simulink model "sysob_simulink"  (R2018b)
settings: Solver=VariableStepAuto  StartTime=0.0  StopTime=10.0  RelTol=1e-3
model workspace: external: MAT-File M:\ParaPower\ARL_ParaPower\Validation\MItest.mat (data not in the file)
values from neighbouring files (symbols this model uses):
  htcs = [1500 1500 500 500 500 500 500 500 500 500]    [MItest.mat]
  Ta_vec = [50 50 50 50 50 50 50 50 50 50]    [MItest.mat]
settings Model: Creator=michael.c.fish  LastModifiedBy=michael.c.fish

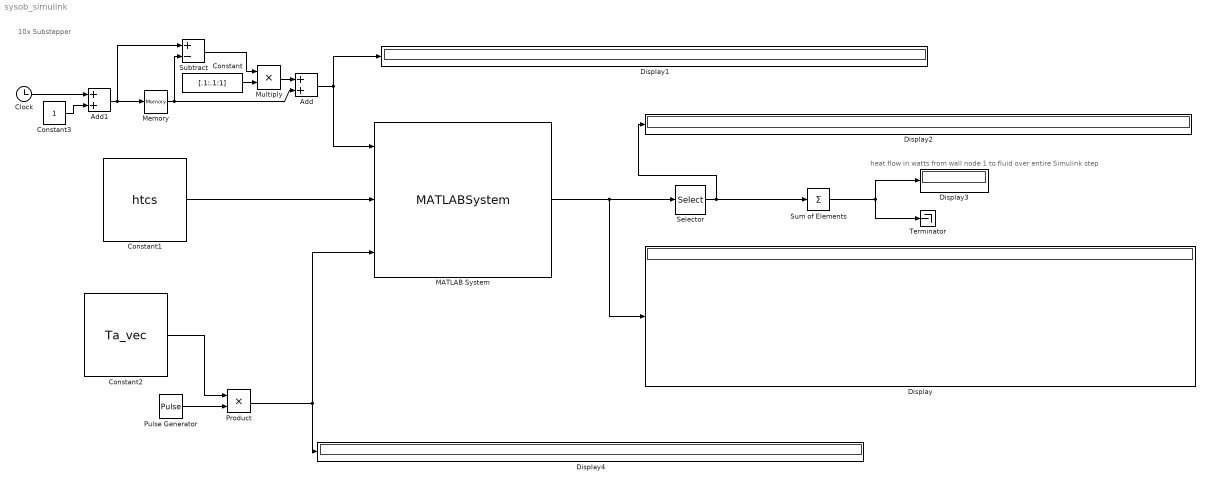
== system sysob_simulink ==
  note: heat flow in watts from wall node 1 to fluid over entire Simulink step
  note: 10x Substepper
  Add : Sum
  Add1 : Sum
  Clock : Clock
  Constant : Constant  Value=[.1:.1:1]  VectorParams1D=off
  Constant1 : Constant  Value=htcs  VectorParams1D=off
  Constant2 : Constant  Value=Ta_vec  VectorParams1D=off
  Constant3 : Constant
  Display{,1..4} (5 alike) : Display
  MATLAB System : MATLABSystem  System=hookPPT  MI=MI  SimulateUsing=Interpreted execution
      mask Type: hookPPT
      mask Display:
      | disp('hookPPT');
      | port_label('input',1,'GlobalTime');
      | port_label('input',2,'htcs');
      | port_label('input',3,'Ta_vec');
      | port_label('output',1,'bdry_watts');
  Memory : Memory
  Multiply : Product
  Product : Product
  Pulse Generator : DiscretePulseGenerator  PulseType=Time based  Period=10  PulseWidth=50
  Selector : Selector  NumberOfDimensions=2  InputPortWidth=3  IndexOptions=Index vector (dialog),Select all  Indices=1,1  OutputSizes=1,1
  Subtract : Sum  Inputs=+-
  Sum of Elements : Sum  Inputs=+
  Terminator : Terminator
  wires:
  Constant1/1 -> MATLAB System/2
  MATLAB System/1 -> Display/1, Selector/1
  Selector/1 -> Sum of Elements/1, Display2/1
  Pulse Generator/1 -> Product/2
  Constant2/1 -> Product/1
  Product/1 -> MATLAB System/3, Display4/1
  Memory/1 -> Add/2, Subtract/2
  Subtract/1 -> Multiply/1
  Constant/1 -> Multiply/2
  Multiply/1 -> Add/1
  Add/1 -> MATLAB System/1, Display1/1
  Add1/1 -> Subtract/1, Memory/1
  Clock/1 -> Add1/1
  Constant3/1 -> Add1/2
  Sum of Elements/1 -> Terminator/1, Display3/1
